simulink model "calibrazione"  (Simulink 7.7)
settings: Solver=ode45  StartTime=0.0  StopTime=10.0  RelTol=1e-3
undefined symbols (not defined in the file): aerosimlib, Earth, WGS
settings Model: Creator=Fede  LastModifiedBy=Fede
settings OptimizationCC: OptimizeModelRefInitCode=on  LifeSpan=1
settings RTWCC: SystemTargetFile=ert.tlc  TemplateMakefile=ert_default_tmf  Description=Embedded Coder  ProcessScript=ert_make_rtw_hook
settings CodeAppCC: IgnoreCustomStorageClasses=off
settings ERTTargetCC: FunctionExecutionProfile=off  MultiwordLength=2048  GenerateSampleERTMain=on  ERTCustomFileTemplate=example_file_process.tlc  ConvertIfToSwitch=off

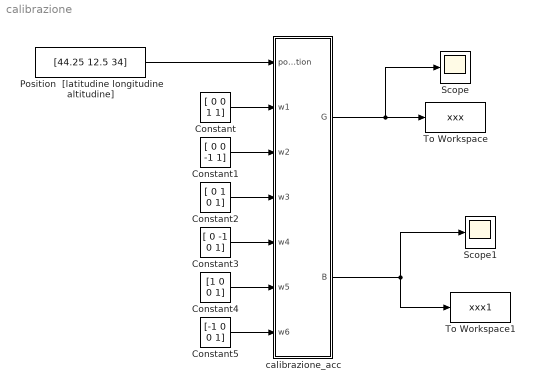
== system calibrazione ==
  Constant : Constant  Value=[ 0 0 1 1]
  Constant1 : Constant  Value=[ 0 0 -1 1]
  Constant2 : Constant  Value=[ 0 1 0 1]
  Constant3 : Constant  Value=[ 0 -1 0 1]
  Constant4 : Constant  Value=[1 0 0 1]
  Constant5 : Constant  Value=[-1 0 0 1]
  Position  [latitudine longitudine altitudine] : Constant  Value=[44.25 12.5 34]
  Scope : Scope
  Scope1 : Scope
  To Workspace : ToWorkspace  VariableName=xxx  SampleTime=-1  SaveFormat=Array
  To Workspace1 : ToWorkspace  VariableName=xxx1  SampleTime=-1  SaveFormat=Array
  calibrazione_acc : Subsystem
  wires:
  Constant/1 -> calibrazione_acc/2(w1)
  Constant1/1 -> calibrazione_acc/3(w2)
  Constant2/1 -> calibrazione_acc/4(w3)
  Constant3/1 -> calibrazione_acc/5(w4)
  Constant4/1 -> calibrazione_acc/6(w5)
  Constant5/1 -> calibrazione_acc/7(w6)
  calibrazione_acc/1(G) -> Scope/1, To Workspace/1
  calibrazione_acc/2(B) -> To Workspace1/1, Scope1/1
  Position  [latitudine longitudine altitudine]/1 -> calibrazione_acc/1(position)

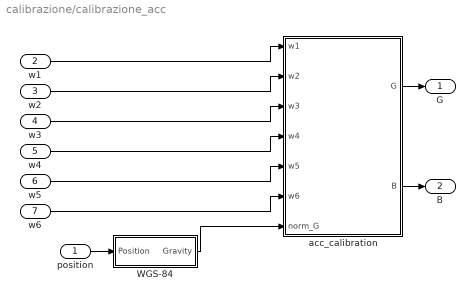
== system calibrazione/calibrazione_acc ==
  position : Inport
  w1 : Inport  Port=2
  w2 : Inport  Port=3
  w3 : Inport  Port=4
  w4 : Inport  Port=5
  w5 : Inport  Port=6
  w6 : Inport  Port=7
  WGS-84 : Subsystem  AncestorBlock=aerosimlib/Earth/WGS-84
      mask Type: WGS-84 Earth model
      mask Description: The WGS-84 Earth model provides local Earth radii and gravity as a function of position.
      mask Help:
      | The block provides a WGS-84 geoid model of the Earth.
      | <P><B>Inputs:</B>
      | <LI>Position = current aircraft location [Latitude Longitude Altitude], in [rad rad m]</LI>
      | </P>
      | <P><B>Output:</B>
      | <LI>Rmeridian = the Earth meridian radius, in m</LI>
      | <LI>Rnormal = the Earth normal radius, in m</LI>
      | <LI>Re = the Earth equivalent radius, in m</LI>
      | <LI>Gravity = the normal gravity, in m/s^2</LI>
      | </P>
  acc_calibration : Stateflow chart  TreatAsAtomicUnit=on
  G : Outport
  B : Outport  Port=2
  wires:
  position/1 -> WGS-84/1(Position)
  w1/1 -> acc_calibration/1(w1)
  w2/1 -> acc_calibration/2(w2)
  acc_calibration/1(G) -> G/1
  w3/1 -> acc_calibration/3(w3)
  w4/1 -> acc_calibration/4(w4)
  w5/1 -> acc_calibration/5(w5)
  acc_calibration/2(B) -> B/1
  w6/1 -> acc_calibration/6(w6)
  WGS-84/1(Gravity) -> acc_calibration/7(norm_G)

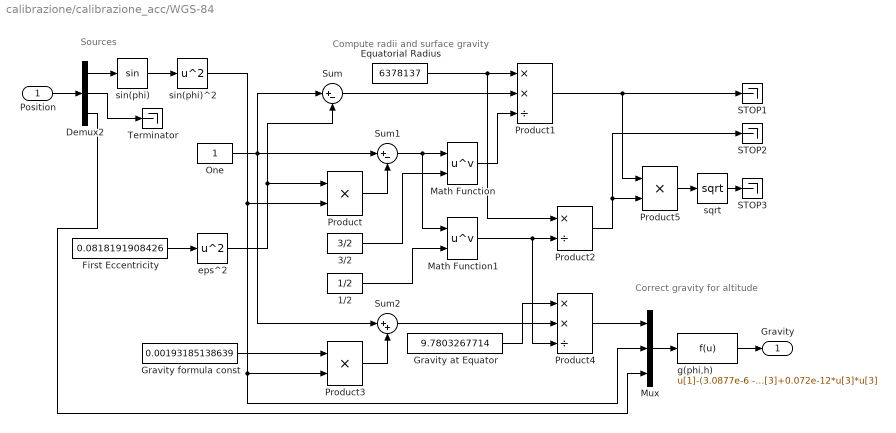
== system calibrazione/calibrazione_acc/WGS-84 ==
  note: Correct gravity for altitude
  note: Compute radii and surface gravity
  note: Sources
  Position : Inport
  1/2 : Constant  Value=1/2
  3/2 : Constant  Value=3/2
  Demux2 : Demux  Outputs=3
  Equatorial Radius : Constant  Value=6378137
  First Eccentricity : Constant  Value=0.0818191908426
  Gravity at Equator : Constant  Value=9.7803267714
  Gravity formula const : Constant  Value=0.00193185138639
  Math Function : Math  Operator=pow  SaturateOnIntegerOverflow=on
  Math Function1 : Math  Operator=pow  SaturateOnIntegerOverflow=on
  Mux : Mux  Inputs=3
  One : Constant
  Product : Product  SaturateOnIntegerOverflow=on  InputSameDT=on  OutDataTypeStr=Inherit: Same as first input
  Product1 : Product  Inputs=**/  SaturateOnIntegerOverflow=on  InputSameDT=on  OutDataTypeStr=Inherit: Same as first input
  Product2 : Product  Inputs=*/  SaturateOnIntegerOverflow=on  InputSameDT=on  OutDataTypeStr=Inherit: Same as first input
  Product3 : Product  SaturateOnIntegerOverflow=on  InputSameDT=on  OutDataTypeStr=Inherit: Same as first input
  Product4 : Product  Inputs=**/  SaturateOnIntegerOverflow=on  InputSameDT=on  OutDataTypeStr=Inherit: Same as first input
  Product5 : Product  SaturateOnIntegerOverflow=on  InputSameDT=on  OutDataTypeStr=Inherit: Same as first input
  STOP1 : Terminator
  STOP2 : Terminator
  STOP3 : Terminator
  Sum : Sum  Inputs=|+-  SaturateOnIntegerOverflow=on  InputSameDT=on  OutDataTypeStr=Inherit: Same as first input
  Sum1 : Sum  Inputs=|+-  SaturateOnIntegerOverflow=on  InputSameDT=on  OutDataTypeStr=Inherit: Same as first input
  Sum2 : Sum  Inputs=|++  SaturateOnIntegerOverflow=on  InputSameDT=on  OutDataTypeStr=Inherit: Same as first input
  Terminator : Terminator
  eps^2 : Math  Operator=square  SaturateOnIntegerOverflow=on
  g(phi,h) : Fcn  Expr=u[1]-(3.0877e-6 - 0.0044e-6*u[2])*u[3]+0.072e-12*u[3]*u[3]
  sin(phi) : Trigonometry
  sin(phi)^2 : Math  Operator=square  SaturateOnIntegerOverflow=on
  sqrt : Math  Operator=sqrt  SaturateOnIntegerOverflow=on
  Gravity : Outport
  wires:
  Demux2/3 -> Mux/3
  g(phi,h)/1 -> Gravity/1
  Mux/1 -> g(phi,h)/1
  Demux2/2 -> Terminator/1
  Demux2/1 -> sin(phi)/1
  Position/1 -> Demux2/1
  Product4/1 -> Mux/1
  Sum2/1 -> Product4/2
  Gravity at Equator/1 -> Product4/1
  Product3/1 -> Sum2/2
  Gravity formula const/1 -> Product3/1
  Product2/1 -> Product5/2, STOP2/1
  Product1/1 -> Product5/1, STOP1/1
  Math Function1/1 -> Product4/3, Product2/2
  Math Function/1 -> Product1/3
  Sum/1 -> Product1/2
  Equatorial Radius/1 -> Product2/1, Product1/1
  1/2/1 -> Math Function1/2
  3/2/1 -> Math Function/2
  Sum1/1 -> Math Function1/1, Math Function/1
  Product/1 -> Sum1/2
  One/1 -> Sum/1, Sum2/1, Sum1/1
  sin(phi)^2/1 -> Mux/2, Product3/2, Product/2
  sin(phi)/1 -> sin(phi)^2/1
  eps^2/1 -> Product/1, Sum/2
  First Eccentricity/1 -> eps^2/1
  Product5/1 -> sqrt/1
  sqrt/1 -> STOP3/1

== matlab function calibrazione_acc/acc_calibration ==
  data: w1 input double; G output double; w2 input double; w3 input double; w4 input double; w5 input double; w6 input double; B output double; norm_G input double
function [G, B] = fcn(w1,w2,w3,w4,w5,w6,norm_G)
%#codegen
Y=[ 0 ,0 ,norm_G;
    0 ,0, -norm_G;
    0 ,norm_G ,0;
    0, -norm_G, 0;
    norm_G ,0 ,0;
    -norm_G ,0, 0];

W=[w1,w2,w3,w4,w5,w6]';
X=((inv(W'*W))*W')*Y;
G=[X(1,1),X(1,2),X(1,3);
    X(2,1),X(2,2),X(2,3);
    X(3,1),X(3,2),X(3,3)];
B=[X(4,1),X(4,2),X(4,3)];
%X=(inv(W'*W))*W'*Y;
